simulink model "fft_26mm_0mm"  (R2020b)
settings: Solver=ode4  StartTime=0.0  StopTime=2  FixedStep=0.000002  RelTol=1e-3
settings Model: Creator=sheikhsoliha  LastModifiedBy=sheikhsoliha
settings DataIOCC: ReturnWorkspaceOutputs=off
settings DebuggingCC: UnconnectedInputMsg=none  UnconnectedOutputMsg=none  UnconnectedLineMsg=none
settings ModelReferenceCC: EnableRefExpFcnMdlSchedulingChecks=off

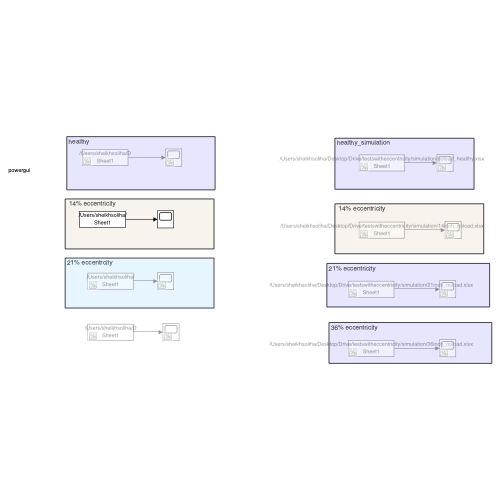
[thumbnail: Simulink's stored preview of the top-level diagram]
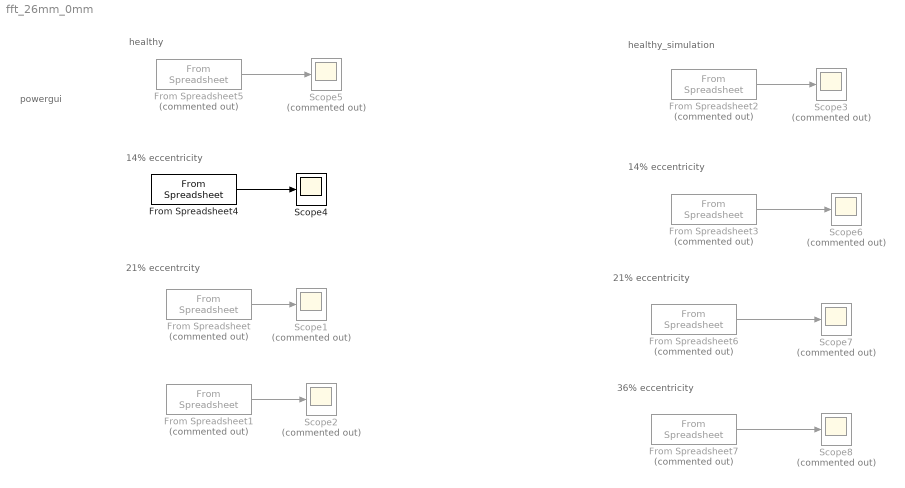
== system fft_26mm_0mm ==
  note: powergui
  note: 36% eccentricity
  note: 21% eccentricity
  note: healthy_simulation
  note: 14% eccentricity
  note: healthy
  note: 21% eccentrcity
  note: 14% eccentricity
  From Spreadsheet : FromSpreadsheet  Commented=on  FileName=/Users/sheikhsoliha/Desktop/Drive/testswitheccentricity/day2_sept6tests/organized/Stator Current/eccentricity_21inch/noload/noload_21inch_morecycles_newer.xlsx
  From Spreadsheet1 : FromSpreadsheet  Commented=on  FileName=/Users/sheikhsoliha/Desktop/Drive/testswitheccentricity/day1_sept5test/Stator Current/eccentricity/noload_0.9398mm/0.9398mm_expt.xlsx
  From Spreadsheet2 : FromSpreadsheet  Commented=on  FileName=/Users/sheikhsoliha/Desktop/Drive/testswitheccentricity/simulation/noload_healthy.xlsx
  From Spreadsheet3 : FromSpreadsheet  Commented=on  FileName=/Users/sheikhsoliha/Desktop/Drive/testswitheccentricity/simulation/14inch_noload.xlsx
  From Spreadsheet4 : FromSpreadsheet  FileName=/Users/sheikhsoliha/Desktop/Paper/FEA /Loading/No Load/-17% & 57% IE/currents for prediction equation/1.3206mm.xlsx  SampleTime=-1
  From Spreadsheet5 : FromSpreadsheet  Commented=on  FileName=/Users/sheikhsoliha/Desktop/Drive/testswitheccentricity/day1_sept5test/Stator Current/noload/noload_expt.xlsx
  From Spreadsheet6 : FromSpreadsheet  Commented=on  FileName=/Users/sheikhsoliha/Desktop/Drive/testswitheccentricity/simulation/21inch_noload.xlsx
  From Spreadsheet7 : FromSpreadsheet  Commented=on  FileName=/Users/sheikhsoliha/Desktop/Drive/testswitheccentricity/simulation/36inch_noload.xlsx
  Scope{1..3,5..8} (7 alike) : Scope  Commented=on
  Scope4 : Scope
  wires:
  From Spreadsheet4/1 -> Scope4/1
  From Spreadsheet5/1 -> Scope5/1
  From Spreadsheet/1 -> Scope1/1
  From Spreadsheet1/1 -> Scope2/1
  From Spreadsheet2/1 -> Scope3/1
  From Spreadsheet3/1 -> Scope6/1
  From Spreadsheet6/1 -> Scope7/1
  From Spreadsheet7/1 -> Scope8/1
